simulink model "serial_comms_test2"  (R2018b)
settings: Solver=ode4  StartTime=0.0  StopTime=100  FixedStep=0.001  RelTol=1e-3
undefined symbols (not defined in the file): serial
libraries: instrumentlib x3
settings Model: EnablePacing=on  Creator=Jared  LastModifiedBy=Jared

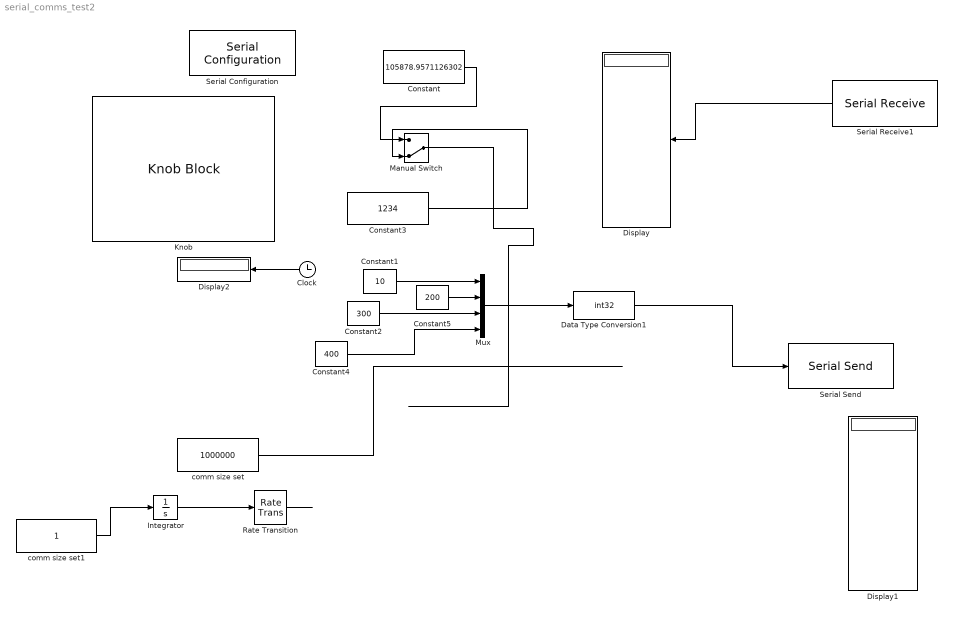
== system serial_comms_test2 ==
  Clock : Clock
  Constant : Constant  Value=105878.9571126302  OutDataTypeStr=double  SampleTime=0.5
  Constant1 : Constant  Value=10  OutDataTypeStr=double  SampleTime=0.5
  Constant2 : Constant  Value=300  OutDataTypeStr=double  SampleTime=0.5
  Constant3 : Constant  Value=1234  OutDataTypeStr=double  SampleTime=0.5
  Constant4 : Constant  Value=400  OutDataTypeStr=double  SampleTime=0.5
  Constant5 : Constant  Value=200  OutDataTypeStr=double  SampleTime=0.5
  Data Type Conversion1 : DataTypeConversion  OutDataTypeStr=int32
  Display : Display
  Display1 : Display
  Display2 : Display
  Integrator : Integrator
  Knob : KnobBlock  WebBlockId=8  ScaleMax=200000
  Manual Switch : ManualSwitch  CurrentSetting=0
  Mux : Mux
  Rate Transition : RateTransition  OutPortSampleTime=1
  Serial Configuration : instrumentlib/Serial Configuration  Priority=-200000  ComPortMenu=<Please select a port...>  ComPort=COM4  ObjConstructor=serial('COM4');  BaudRate=9600  DataBits=8  Parity=none  StopBits=1  FlowControl=none  Timeout=10  ByteOrder=LittleEndian
  Serial Receive1 : instrumentlib/Serial Receive  ComPortMenu=<Please select a port...>  ComPort=COM4  ObjConstructor=serial('COM4');  Header=\n  Terminator=\n  DataSize="[4  1]"  DataType=uint32  EnableBlockingMode=on  ActionDataUnavailable=Output last received value  CustomValue=0  SampleTime=1.5
  Serial Send : instrumentlib/Serial Send  ComPortMenu=<Please select a port...>  ComPort=COM4  ObjConstructor=serial('COM4');  Terminator=<none>  EnableBlockingMode=on
  comm size set : Constant  Value=1000000  OutDataTypeStr=double  SampleTime=0.5
  comm size set1 : Constant  OutDataTypeStr=double  SampleTime=0.5
  wires:
  Clock/1 -> Display2/1
  Mux/1 -> Data Type Conversion1/1
  Constant1/1 -> Mux/1
  Manual Switch/1 -> ?
  Constant3/1 -> Manual Switch/2
  Constant/1 -> Manual Switch/1
  Data Type Conversion1/1 -> Serial Send/1
  Serial Receive1/1 -> Display/1
  comm size set/1 -> ?
  comm size set1/1 -> Integrator/1
  Integrator/1 -> Rate Transition/1
  Rate Transition/1 -> ?
  Constant4/1 -> Mux/4
  Constant2/1 -> Mux/3
  Constant5/1 -> Mux/2
